simulink model "PeakDetect_500"  (R2018b)
settings: Solver=FixedStepAuto  StartTime=0  StopTime=500*(15e-9)  FixedStep=15e-9  RelTol=1e-3
libraries: simulink x35, hdlsllib x34
(part 3 of 3)

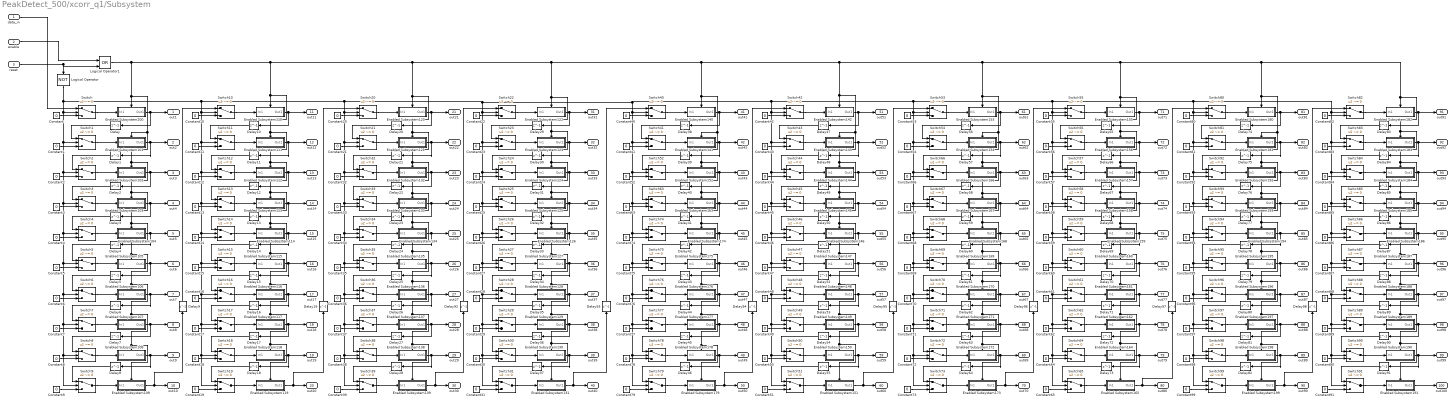
== system PeakDetect_500/xcorr_q1/Subsystem ==
  data_in : Inport  OutDataTypeStr=fixdt(1,16,15)
  enable : Inport  Port=2
  reset : Inport  Port=3
  Constant{,1..99} (100 alike) : Constant  Value=0  OutDataTypeStr=Inherit: Inherit via back propagation  SampleTime=-1
  Delay{,1..98} (99 alike) : Delay  DelayLength=1
  Enabled Subsystem101 : Subsystem  TreatAsAtomicUnit=on
  Enabled Subsystem102 : Subsystem  TreatAsAtomicUnit=on
  Enabled Subsystem103 : Subsystem  TreatAsAtomicUnit=on
  Enabled Subsystem104 : Subsystem  TreatAsAtomicUnit=on
  Enabled Subsystem105 : Subsystem  TreatAsAtomicUnit=on
  Enabled Subsystem106 : Subsystem  TreatAsAtomicUnit=on
  Enabled Subsystem107 : Subsystem  TreatAsAtomicUnit=on
  Enabled Subsystem108 : Subsystem  TreatAsAtomicUnit=on
  Enabled Subsystem109 : Subsystem  TreatAsAtomicUnit=on
  Enabled Subsystem110 : Subsystem  TreatAsAtomicUnit=on
  Enabled Subsystem111 : Subsystem  TreatAsAtomicUnit=on
  Enabled Subsystem112 : Subsystem  TreatAsAtomicUnit=on
  Enabled Subsystem113 : Subsystem  TreatAsAtomicUnit=on
  Enabled Subsystem114 : Subsystem  TreatAsAtomicUnit=on
  Enabled Subsystem115 : Subsystem  TreatAsAtomicUnit=on
  Enabled Subsystem116 : Subsystem  TreatAsAtomicUnit=on
  Enabled Subsystem117 : Subsystem  TreatAsAtomicUnit=on
  Enabled Subsystem118 : Subsystem  TreatAsAtomicUnit=on
  Enabled Subsystem119 : Subsystem  TreatAsAtomicUnit=on
  Enabled Subsystem120 : Subsystem  TreatAsAtomicUnit=on
  Enabled Subsystem121 : Subsystem  TreatAsAtomicUnit=on
  Enabled Subsystem122 : Subsystem  TreatAsAtomicUnit=on
  Enabled Subsystem123 : Subsystem  TreatAsAtomicUnit=on
  Enabled Subsystem124 : Subsystem  TreatAsAtomicUnit=on
  Enabled Subsystem125 : Subsystem  TreatAsAtomicUnit=on
  Enabled Subsystem126 : Subsystem  TreatAsAtomicUnit=on
  Enabled Subsystem127 : Subsystem  TreatAsAtomicUnit=on
  Enabled Subsystem128 : Subsystem  TreatAsAtomicUnit=on
  Enabled Subsystem129 : Subsystem  TreatAsAtomicUnit=on
  Enabled Subsystem130 : Subsystem  TreatAsAtomicUnit=on
  Enabled Subsystem131 : Subsystem  TreatAsAtomicUnit=on
  Enabled Subsystem132 : Subsystem  TreatAsAtomicUnit=on
  Enabled Subsystem133 : Subsystem  TreatAsAtomicUnit=on
  Enabled Subsystem134 : Subsystem  TreatAsAtomicUnit=on
  Enabled Subsystem135 : Subsystem  TreatAsAtomicUnit=on
  Enabled Subsystem136 : Subsystem  TreatAsAtomicUnit=on
  Enabled Subsystem137 : Subsystem  TreatAsAtomicUnit=on
  Enabled Subsystem138 : Subsystem  TreatAsAtomicUnit=on
  Enabled Subsystem139 : Subsystem  TreatAsAtomicUnit=on
  Enabled Subsystem140 : Subsystem  TreatAsAtomicUnit=on
  Enabled Subsystem141 : Subsystem  TreatAsAtomicUnit=on
  Enabled Subsystem142 : Subsystem  TreatAsAtomicUnit=on
  Enabled Subsystem143 : Subsystem  TreatAsAtomicUnit=on
  Enabled Subsystem144 : Subsystem  TreatAsAtomicUnit=on
  Enabled Subsystem145 : Subsystem  TreatAsAtomicUnit=on
  Enabled Subsystem146 : Subsystem  TreatAsAtomicUnit=on
  Enabled Subsystem147 : Subsystem  TreatAsAtomicUnit=on
  Enabled Subsystem148 : Subsystem  TreatAsAtomicUnit=on
  Enabled Subsystem149 : Subsystem  TreatAsAtomicUnit=on
  Enabled Subsystem150 : Subsystem  TreatAsAtomicUnit=on
  Enabled Subsystem151 : Subsystem  TreatAsAtomicUnit=on
  Enabled Subsystem152 : Subsystem  TreatAsAtomicUnit=on
  Enabled Subsystem153 : Subsystem  TreatAsAtomicUnit=on
  Enabled Subsystem154 : Subsystem  TreatAsAtomicUnit=on
  Enabled Subsystem155 : Subsystem  TreatAsAtomicUnit=on
  Enabled Subsystem156 : Subsystem  TreatAsAtomicUnit=on
  Enabled Subsystem157 : Subsystem  TreatAsAtomicUnit=on
  Enabled Subsystem158 : Subsystem  TreatAsAtomicUnit=on
  Enabled Subsystem159 : Subsystem  TreatAsAtomicUnit=on
  Enabled Subsystem160 : Subsystem  TreatAsAtomicUnit=on
  Enabled Subsystem161 : Subsystem  TreatAsAtomicUnit=on
  Enabled Subsystem162 : Subsystem  TreatAsAtomicUnit=on
  Enabled Subsystem163 : Subsystem  TreatAsAtomicUnit=on
  Enabled Subsystem164 : Subsystem  TreatAsAtomicUnit=on
  Enabled Subsystem165 : Subsystem  TreatAsAtomicUnit=on
  Enabled Subsystem166 : Subsystem  TreatAsAtomicUnit=on
  Enabled Subsystem167 : Subsystem  TreatAsAtomicUnit=on
  Enabled Subsystem168 : Subsystem  TreatAsAtomicUnit=on
  Enabled Subsystem169 : Subsystem  TreatAsAtomicUnit=on
  Enabled Subsystem170 : Subsystem  TreatAsAtomicUnit=on
  Enabled Subsystem171 : Subsystem  TreatAsAtomicUnit=on
  Enabled Subsystem172 : Subsystem  TreatAsAtomicUnit=on
  Enabled Subsystem173 : Subsystem  TreatAsAtomicUnit=on
  Enabled Subsystem174 : Subsystem  TreatAsAtomicUnit=on
  Enabled Subsystem175 : Subsystem  TreatAsAtomicUnit=on
  Enabled Subsystem176 : Subsystem  TreatAsAtomicUnit=on
  Enabled Subsystem177 : Subsystem  TreatAsAtomicUnit=on
  Enabled Subsystem178 : Subsystem  TreatAsAtomicUnit=on
  Enabled Subsystem179 : Subsystem  TreatAsAtomicUnit=on
  Enabled Subsystem180 : Subsystem  TreatAsAtomicUnit=on
  Enabled Subsystem181 : Subsystem  TreatAsAtomicUnit=on
  Enabled Subsystem182 : Subsystem  TreatAsAtomicUnit=on
  Enabled Subsystem183 : Subsystem  TreatAsAtomicUnit=on
  Enabled Subsystem184 : Subsystem  TreatAsAtomicUnit=on
  Enabled Subsystem185 : Subsystem  TreatAsAtomicUnit=on
  Enabled Subsystem186 : Subsystem  TreatAsAtomicUnit=on
  Enabled Subsystem187 : Subsystem  TreatAsAtomicUnit=on
  Enabled Subsystem188 : Subsystem  TreatAsAtomicUnit=on
  Enabled Subsystem189 : Subsystem  TreatAsAtomicUnit=on
  Enabled Subsystem190 : Subsystem  TreatAsAtomicUnit=on
  Enabled Subsystem191 : Subsystem  TreatAsAtomicUnit=on
  Enabled Subsystem192 : Subsystem  TreatAsAtomicUnit=on
  Enabled Subsystem193 : Subsystem  TreatAsAtomicUnit=on
  Enabled Subsystem194 : Subsystem  TreatAsAtomicUnit=on
  Enabled Subsystem195 : Subsystem  TreatAsAtomicUnit=on
  Enabled Subsystem196 : Subsystem  TreatAsAtomicUnit=on
  Enabled Subsystem197 : Subsystem  TreatAsAtomicUnit=on
  Enabled Subsystem198 : Subsystem  TreatAsAtomicUnit=on
  Enabled Subsystem199 : Subsystem  TreatAsAtomicUnit=on
  Enabled Subsystem200 : Subsystem  TreatAsAtomicUnit=on
  Logical Operator : Logic  Operator=NOT  IconShape=distinctive  AllPortsSameDT=off  OutDataTypeStr=boolean
  Logical Operator1 : Logic  Operator=OR  IconShape=distinctive  AllPortsSameDT=off  OutDataTypeStr=boolean
  Switch{,1..99} (100 alike) : Switch  Criteria=u2 ~= 0  OutDataTypeStr=Inherit: Inherit via back propagation
  out1 : Outport
  out2 : Outport  Port=2
  out3 : Outport  Port=3
  out4 : Outport  Port=4
  out5 : Outport  Port=5
  out6 : Outport  Port=6
  out7 : Outport  Port=7
  out8 : Outport  Port=8
  out9 : Outport  Port=9
  out10 : Outport  Port=10
  out11 : Outport  Port=11
  out12 : Outport  Port=12
  out13 : Outport  Port=13
  out14 : Outport  Port=14
  out15 : Outport  Port=15
  out16 : Outport  Port=16
  out17 : Outport  Port=17
  out18 : Outport  Port=18
  out19 : Outport  Port=19
  out20 : Outport  Port=20
  out21 : Outport  Port=21
  out22 : Outport  Port=22
  out23 : Outport  Port=23
  out24 : Outport  Port=24
  out25 : Outport  Port=25
  out26 : Outport  Port=26
  out27 : Outport  Port=27
  out28 : Outport  Port=28
  out29 : Outport  Port=29
  out30 : Outport  Port=30
  out31 : Outport  Port=31
  out32 : Outport  Port=32
  out33 : Outport  Port=33
  out34 : Outport  Port=34
  out35 : Outport  Port=35
  out36 : Outport  Port=36
  out37 : Outport  Port=37
  out38 : Outport  Port=38
  out39 : Outport  Port=39
  out40 : Outport  Port=40
  out41 : Outport  Port=41
  out42 : Outport  Port=42
  out43 : Outport  Port=43
  out44 : Outport  Port=44
  out45 : Outport  Port=45
  out46 : Outport  Port=46
  out47 : Outport  Port=47
  out48 : Outport  Port=48
  out49 : Outport  Port=49
  out50 : Outport  Port=50
  out51 : Outport  Port=51
  out52 : Outport  Port=52
  out53 : Outport  Port=53
  out54 : Outport  Port=54
  out55 : Outport  Port=55
  out56 : Outport  Port=56
  out57 : Outport  Port=57
  out58 : Outport  Port=58
  out59 : Outport  Port=59
  out60 : Outport  Port=60
  out61 : Outport  Port=61
  out62 : Outport  Port=62
  out63 : Outport  Port=63
  out64 : Outport  Port=64
  out65 : Outport  Port=65
  out66 : Outport  Port=66
  out67 : Outport  Port=67
  out68 : Outport  Port=68
  out69 : Outport  Port=69
  out70 : Outport  Port=70
  out71 : Outport  Port=71
  out72 : Outport  Port=72
  out73 : Outport  Port=73
  out74 : Outport  Port=74
  out75 : Outport  Port=75
  out76 : Outport  Port=76
  out77 : Outport  Port=77
  out78 : Outport  Port=78
  out79 : Outport  Port=79
  out80 : Outport  Port=80
  out81 : Outport  Port=81
  out82 : Outport  Port=82
  out83 : Outport  Port=83
  out84 : Outport  Port=84
  out85 : Outport  Port=85
  out86 : Outport  Port=86
  out87 : Outport  Port=87
  out88 : Outport  Port=88
  out89 : Outport  Port=89
  out90 : Outport  Port=90
  out91 : Outport  Port=91
  out92 : Outport  Port=92
  out93 : Outport  Port=93
  out94 : Outport  Port=94
  out95 : Outport  Port=95
  out96 : Outport  Port=96
  out97 : Outport  Port=97
  out98 : Outport  Port=98
  out99 : Outport  Port=99
  out100 : Outport  Port=100
  wires:
  Delay81/1 -> Switch98/1
  Delay36/1 -> Switch30/1
  Constant37/1 -> Switch37/3
  Switch72/1 -> Enabled Subsystem172/1(In1)
  Switch33/1 -> Enabled Subsystem133/1(In1)
  Delay65/1 -> Switch56/1
  Constant39/1 -> Switch39/3
  Switch76/1 -> Enabled Subsystem176/1(In1)
  Constant59/1 -> Switch59/3
  Constant70/1 -> Switch70/3
  Constant12/1 -> Switch12/3
  Constant58/1 -> Switch58/3
  Delay52/1 -> Switch48/1
  Switch58/1 -> Enabled Subsystem158/1(In1)
  Constant55/1 -> Switch55/3
  Switch29/1 -> Enabled Subsystem129/1(In1)
  Switch37/1 -> Enabled Subsystem137/1(In1)
  Constant99/1 -> Switch99/3
  Constant22/1 -> Switch22/3
  Constant34/1 -> Switch34/3
  Switch38/1 -> Enabled Subsystem138/1(In1)
  Delay/1 -> Switch1/1
  Switch23/1 -> Enabled Subsystem123/1(In1)
  Delay25/1 -> Switch36/1
  Delay22/1 -> Switch33/1
  Delay50/1 -> Switch46/1
  Constant53/1 -> Switch53/3
  Enabled Subsystem197/1(Out1) -> out88/1, Delay81/1
  Switch45/1 -> Enabled Subsystem145/1(In1)
  Switch6/1 -> Enabled Subsystem106/1(In1)
  Delay92/1 -> Switch22/1
  Switch55/1 -> Enabled Subsystem155/1(In1)
  Constant38/1 -> Switch38/3
  Delay58/1 -> Switch67/1
  Enabled Subsystem176/1(Out1) -> out47/1, Delay44/1
  Constant54/1 -> Switch54/3
  Constant31/1 -> Switch31/3
  Enabled Subsystem139/1(Out1) -> out30/1, Delay92/1
  Delay94/1 -> Switch42/1
  Switch90/1 -> Enabled Subsystem190/1(In1)
  Delay8/1 -> Switch9/1
  Constant50/1 -> Switch50/3
  Enabled Subsystem155/1(Out1) -> out71/1, Delay65/1
  Delay72/1 -> Switch64/1
  Constant76/1 -> Switch76/3
  Switch73/1 -> Enabled Subsystem173/1(In1)
  Constant41/1 -> Switch41/3
  Constant97/1 -> Switch97/3
  Switch44/1 -> Enabled Subsystem144/1(In1)
  Switch77/1 -> Enabled Subsystem177/1(In1)
  Constant47/1 -> Switch47/3
  Constant62/1 -> Switch62/3
  Switch3/1 -> Enabled Subsystem103/1(In1)
  Constant71/1 -> Switch71/3
  Delay37/1 -> Switch31/1
  Constant75/1 -> Switch75/3
  Constant93/1 -> Switch93/3
  Switch2/1 -> Enabled Subsystem102/1(In1)
  Constant29/1 -> Switch29/3
  Enabled Subsystem172/1(Out1) -> out69/1, Delay64/1
  Delay24/1 -> Switch35/1
  Constant56/1 -> Switch56/3
  Switch8/1 -> Enabled Subsystem108/1(In1)
  Switch31/1 -> Enabled Subsystem131/1(In1)
  Delay89/1 -> Switch89/1
  Delay27/1 -> Switch38/1
  Constant2/1 -> Switch2/3
  Switch13/1 -> Enabled Subsystem113/1(In1)
  Constant/1 -> Switch/3
  Delay64/1 -> Switch73/1
  Constant81/1 -> Switch81/3
  Constant40/1 -> Switch40/3
  Switch52/1 -> Enabled Subsystem152/1(In1)
  Switch14/1 -> Enabled Subsystem114/1(In1)
  Enabled Subsystem117/1(Out1) -> out18/1, Delay17/1
  Constant49/1 -> Switch49/3
  Switch70/1 -> Enabled Subsystem170/1(In1)
  Constant64/1 -> Switch64/3
  Switch82/1 -> Enabled Subsystem182/1(In1)
  Delay98/1 -> Switch82/1
  Enabled Subsystem177/1(Out1) -> out48/1, Delay45/1
  Enabled Subsystem159/1(Out1) -> out75/1, Delay69/1
  Constant68/1 -> Switch68/3
  Enabled Subsystem101/1(Out1) -> out2/1, Delay1/1
  Constant92/1 -> Switch92/3
  Enabled Subsystem152/1(Out1) -> out43/1, Delay40/1
  Enabled Subsystem136/1(Out1) -> out27/1, Delay26/1
  Delay86/1 -> Switch86/1
  Constant83/1 -> Switch83/3
  Switch83/1 -> Enabled Subsystem183/1(In1)
  Enabled Subsystem163/1(Out1) -> out44/1, Delay41/1
  Switch15/1 -> Enabled Subsystem115/1(In1)
  Constant46/1 -> Switch46/3
  Delay39/1 -> Switch52/1
  Delay31/1 -> Switch25/1
  Constant6/1 -> Switch6/3
  Switch26/1 -> Enabled Subsystem126/1(In1)
  Delay29/1 -> Switch23/1
  Constant28/1 -> Switch28/3
  Constant11/1 -> Switch11/3
  Constant9/1 -> Switch9/3
  Enabled Subsystem105/1(Out1) -> out6/1, Delay5/1
  Delay48/1 -> Switch44/1
  Switch4/1 -> Enabled Subsystem104/1(In1)
  Delay77/1 -> Switch94/1
  Constant24/1 -> Switch24/3
  Switch17/1 -> Enabled Subsystem117/1(In1)
  Switch32/1 -> Enabled Subsystem132/1(In1)
  Enabled Subsystem149/1(Out1) -> out58/1, Delay54/1
  Constant73/1 -> Switch73/3
  Switch34/1 -> Enabled Subsystem134/1(In1)
  Delay76/1 -> Switch93/1
  Enabled Subsystem148/1(Out1) -> out57/1, Delay53/1
  Switch74/1 -> Enabled Subsystem174/1(In1)
  Enabled Subsystem153/1(Out1) -> out61/1, Delay56/1
  Enabled Subsystem144/1(Out1) -> out53/1, Delay49/1
  Delay90/1 -> Switch90/1
  Constant61/1 -> Switch61/3
  Switch63/1 -> Enabled Subsystem163/1(In1)
  Switch89/1 -> Enabled Subsystem189/1(In1)
  Switch94/1 -> Enabled Subsystem194/1(In1)
  Delay67/1 -> Switch58/1
  Constant19/1 -> Switch19/3
  Switch65/1 -> Enabled Subsystem165/1(In1)
  Constant4/1 -> Switch4/3
  Constant96/1 -> Switch96/3
  Enabled Subsystem167/1(Out1) -> out64/1, Delay59/1
  Delay75/1 -> Switch92/1
  Delay11/1 -> Switch12/1
  Constant51/1 -> Switch51/3
  Enabled Subsystem111/1(Out1) -> out12/1, Delay11/1
  Switch11/1 -> Enabled Subsystem111/1(In1)
  Constant94/1 -> Switch94/3
  Switch28/1 -> Enabled Subsystem128/1(In1)
  Constant80/1 -> Switch80/3
  Constant74/1 -> Switch74/3
  Switch27/1 -> Enabled Subsystem127/1(In1)
  Enabled Subsystem110/1(Out1) -> out11/1, Delay10/1
  Delay97/1 -> Switch80/1
  Enabled Subsystem200/1(Out1) -> out1/1, Delay/1
  Switch95/1 -> Enabled Subsystem195/1(In1)
  Switch99/1 -> Enabled Subsystem199/1(In1)
  Switch12/1 -> Enabled Subsystem112/1(In1)
  Switch19/1 -> Enabled Subsystem119/1(In1)
  Switch36/1 -> Enabled Subsystem136/1(In1)
  Constant87/1 -> Switch87/3
  Delay7/1 -> Switch8/1
  Constant30/1 -> Switch30/3
  Enabled Subsystem150/1(Out1) -> out59/1, Delay55/1
  Switch51/1 -> Enabled Subsystem151/1(In1)
  Constant33/1 -> Switch33/3
  Enabled Subsystem160/1(Out1) -> out76/1, Delay70/1
  Delay28/1 -> Switch39/1
  Enabled Subsystem154/1(Out1) -> out62/1, Delay57/1
  Delay41/1 -> Switch74/1
  Delay3/1 -> Switch4/1
  Constant8/1 -> Switch8/3
  Constant72/1 -> Switch72/3
  Switch61/1 -> Enabled Subsystem161/1(In1)
  Constant18/1 -> Switch18/3
  Delay79/1 -> Switch96/1
  Enabled Subsystem193/1(Out1) -> out84/1, Delay77/1
  Delay88/1 -> Switch88/1
  Constant67/1 -> Switch67/3
  Switch97/1 -> Enabled Subsystem197/1(In1)
  data_in/1 -> Switch/1
  Enabled Subsystem113/1(Out1) -> out14/1, Delay13/1
  Constant82/1 -> Switch82/3
  Constant15/1 -> Switch15/3
  Switch93/1 -> Enabled Subsystem193/1(In1)
  Delay61/1 -> Switch70/1
  Logical Operator/1 -> Switch91/2, Switch90/2, Switch89/2, Switch88/2, Switch87/2, Switch86/2, Switch85/2, Switch84/2, Switch83/2, Switch82/2, Switch99/2, Switch98/2, Switch97/2, Switch96/2, Switch95/2, Switch94/2, Switch93/2, Switch92/2, Switch81/2, Switch80/2, Switch65/2, Switch64/2, Switch62/2, Switch61/2, Switch60/2, Switch59/2, Switch58/2, Switch57/2, Switch56/2, Switch55/2, Switch73/2, Switch72/2, Switch71/2, Switch70/2, Switch69/2, Switch68/2, Switch67/2, Switch66/2, Switch54/2, Switch53/2, Switch51/2, Switch50/2, Switch49/2, Switch48/2, Switch47/2, Switch46/2, Switch45/2, Switch44/2, Switch43/2, Switch42/2, Switch79/2, Switch78/2, Switch77/2, Switch76/2, Switch75/2, Switch74/2, Switch63/2, Switch52/2, Switch41/2, Switch40/2, Switch31/2, Switch30/2, Switch29/2, Switch28/2, Switch27/2, Switch26/2, Switch25/2, Switch24/2, Switch23/2, Switch22/2, Switch39/2, Switch38/2, Switch37/2, Switch36/2, Switch35/2, Switch34/2, Switch33/2, Switch32/2, Switch21/2, Switch20/2, Switch19/2, Switch18/2, Switch17/2, Switch16/2, Switch15/2, Switch14/2, Switch13/2, Switch12/2, Switch11/2, Switch10/2, Switch9/2, Switch8/2, Switch7/2, Switch6/2, Switch5/2, Switch4/2, Switch3/2, Switch2/2, Switch1/2, Switch/2
  Delay85/1 -> Switch85/1
  Switch25/1 -> Enabled Subsystem125/1(In1)
  Enabled Subsystem118/1(Out1) -> out19/1, Delay18/1
  Enabled Subsystem129/1(Out1) -> out38/1, Delay36/1
  Switch80/1 -> Enabled Subsystem180/1(In1)
  Enabled Subsystem112/1(Out1) -> out13/1, Delay12/1
  Enabled Subsystem120/1(Out1) -> out21/1, Delay20/1
  Switch21/1 -> Enabled Subsystem121/1(In1)
  Delay18/1 -> Switch19/1
  Enabled Subsystem134/1(Out1) -> out25/1, Delay24/1
  Enabled Subsystem147/1(Out1) -> out56/1, Delay52/1
  Constant86/1 -> Switch86/3
  Constant35/1 -> Switch35/3
  Delay9/1 -> Switch10/1
  Constant13/1 -> Switch13/3
  Delay93/1 -> Switch40/1
  Enabled Subsystem166/1(Out1) -> out63/1, Delay58/1
  Delay59/1 -> Switch68/1
  Enabled Subsystem157/1(Out1) -> out73/1, Delay67/1
  Switch88/1 -> Enabled Subsystem188/1(In1)
  Constant66/1 -> Switch66/3
  Delay32/1 -> Switch26/1
  Constant88/1 -> Switch88/3
  Enabled Subsystem130/1(Out1) -> out39/1, Delay37/1
  Switch79/1 -> Enabled Subsystem179/1(In1)
  Constant89/1 -> Switch89/3
  Enabled Subsystem161/1(Out1) -> out77/1, Delay71/1
  Delay16/1 -> Switch17/1
  Switch56/1 -> Enabled Subsystem156/1(In1)
  Enabled Subsystem185/1(Out1) -> out94/1, Delay86/1
  Enabled Subsystem164/1(Out1) -> out79/1, Delay73/1
  Delay71/1 -> Switch62/1
  Enabled Subsystem180/1(Out1) -> out81/1, Delay74/1
  Enabled Subsystem171/1(Out1) -> out68/1, Delay63/1
  Enabled Subsystem184/1(Out1) -> out93/1, Delay85/1
  Enabled Subsystem107/1(Out1) -> out8/1, Delay7/1
  Switch75/1 -> Enabled Subsystem175/1(In1)
  Switch18/1 -> Enabled Subsystem118/1(In1)
  Delay38/1 -> Switch41/1
  Constant85/1 -> Switch85/3
  Switch47/1 -> Enabled Subsystem147/1(In1)
  Constant91/1 -> Switch91/3
  Constant26/1 -> Switch26/3
  Delay2/1 -> Switch3/1
  Delay57/1 -> Switch66/1
  Constant20/1 -> Switch20/3
  Delay82/1 -> Switch99/1
  Enabled Subsystem122/1(Out1) -> out31/1, Delay29/1
  Delay70/1 -> Switch61/1
  Delay33/1 -> Switch27/1
  Constant60/1 -> Switch60/3
  Delay95/1 -> Switch53/1
  Constant32/1 -> Switch32/3
  Switch87/1 -> Enabled Subsystem187/1(In1)
  Enabled Subsystem182/1(Out1) -> out91/1, Delay83/1
  Switch92/1 -> Enabled Subsystem192/1(In1)
  Delay13/1 -> Switch14/1
  Delay47/1 -> Switch43/1
  Constant98/1 -> Switch98/3
  Switch81/1 -> Enabled Subsystem181/1(In1)
  Delay96/1 -> Switch55/1
  Delay35/1 -> Switch29/1
  Delay73/1 -> Switch65/1
  Enabled Subsystem196/1(Out1) -> out87/1, Delay80/1
  Enabled Subsystem103/1(Out1) -> out4/1, Delay3/1
  Constant23/1 -> Switch23/3
  Constant90/1 -> Switch90/3
  Enabled Subsystem125/1(Out1) -> out34/1, Delay32/1
  Enabled Subsystem169/1(Out1) -> out66/1, Delay61/1
  Constant78/1 -> Switch78/3
  Constant27/1 -> Switch27/3
  Delay14/1 -> Switch15/1
  Enabled Subsystem104/1(Out1) -> out5/1, Delay4/1
  Constant36/1 -> Switch36/3
  Switch39/1 -> Enabled Subsystem139/1(In1)
  Delay42/1 -> Switch75/1
  Enabled Subsystem114/1(Out1) -> out15/1, Delay14/1
  Enabled Subsystem146/1(Out1) -> out55/1, Delay51/1
  Switch57/1 -> Enabled Subsystem157/1(In1)
  Delay87/1 -> Switch87/1
  Enabled Subsystem137/1(Out1) -> out28/1, Delay27/1
  Constant84/1 -> Switch84/3
  Constant1/1 -> Switch1/3
  Enabled Subsystem173/1(Out1) -> out70/1, Delay96/1
  Switch41/1 -> Enabled Subsystem141/1(In1)
  Delay20/1 -> Switch21/1
  Delay68/1 -> Switch59/1
  Switch98/1 -> Enabled Subsystem198/1(In1)
  Delay43/1 -> Switch76/1
  Constant65/1 -> Switch65/3
  Constant17/1 -> Switch17/3
  Switch60/1 -> Enabled Subsystem160/1(In1)
  Enabled Subsystem162/1(Out1) -> out78/1, Delay72/1
  Constant7/1 -> Switch7/3
  Delay78/1 -> Switch95/1
  Enabled Subsystem191/1(Out1) -> out100/1
  Switch40/1 -> Enabled Subsystem140/1(In1)
  Switch78/1 -> Enabled Subsystem178/1(In1)
  Switch85/1 -> Enabled Subsystem185/1(In1)
  Delay12/1 -> Switch13/1
  Switch86/1 -> Enabled Subsystem186/1(In1)
  Delay84/1 -> Switch84/1
  Constant77/1 -> Switch77/3
  Delay6/1 -> Switch7/1
  Constant42/1 -> Switch42/3
  Delay80/1 -> Switch97/1
  Delay53/1 -> Switch49/1
  Enabled Subsystem128/1(Out1) -> out37/1, Delay35/1
  Enabled Subsystem170/1(Out1) -> out67/1, Delay62/1
  Enabled Subsystem102/1(Out1) -> out3/1, Delay2/1
  Enabled Subsystem194/1(Out1) -> out85/1, Delay78/1
  Constant10/1 -> Switch10/3
  Enabled Subsystem187/1(Out1) -> out96/1, Delay88/1
  enable/1 -> Logical Operator1/1
  Enabled Subsystem123/1(Out1) -> out32/1, Delay30/1
  Delay26/1 -> Switch37/1
  Switch62/1 -> Enabled Subsystem162/1(In1)
  Enabled Subsystem141/1(Out1) -> out42/1, Delay39/1
  Delay83/1 -> Switch83/1
  Delay45/1 -> Switch78/1
  Switch10/1 -> Enabled Subsystem110/1(In1)
  Enabled Subsystem138/1(Out1) -> out29/1, Delay28/1
  Enabled Subsystem192/1(Out1) -> out83/1, Delay76/1
  Delay5/1 -> Switch6/1
  Switch53/1 -> Enabled Subsystem153/1(In1)
  Enabled Subsystem126/1(Out1) -> out35/1, Delay33/1
  Switch48/1 -> Enabled Subsystem148/1(In1)
  Delay55/1 -> Switch51/1
  Delay34/1 -> Switch28/1
  Switch7/1 -> Enabled Subsystem107/1(In1)
  Enabled Subsystem186/1(Out1) -> out95/1, Delay87/1
  Delay10/1 -> Switch11/1
  Enabled Subsystem199/1(Out1) -> out90/1, Delay98/1
  Constant52/1 -> Switch52/3
  Switch96/1 -> Enabled Subsystem196/1(In1)
  Constant44/1 -> Switch44/3
  Delay69/1 -> Switch60/1
  Enabled Subsystem131/1(Out1) -> out40/1, Delay93/1
  Enabled Subsystem179/1(Out1) -> out50/1, Delay94/1
  Switch46/1 -> Enabled Subsystem146/1(In1)
  Delay30/1 -> Switch24/1
  Enabled Subsystem133/1(Out1) -> out24/1, Delay23/1
  Enabled Subsystem109/1(Out1) -> out10/1, Delay9/1
  Enabled Subsystem119/1(Out1) -> out20/1, Delay19/1
  Switch5/1 -> Enabled Subsystem105/1(In1)
  Constant69/1 -> Switch69/3
  Enabled Subsystem142/1(Out1) -> out51/1, Delay47/1
  Delay17/1 -> Switch18/1
  Constant45/1 -> Switch45/3
  Delay46/1 -> Switch79/1
  Enabled Subsystem181/1(Out1) -> out82/1, Delay75/1
  Enabled Subsystem135/1(Out1) -> out26/1, Delay25/1
  Enabled Subsystem124/1(Out1) -> out33/1, Delay31/1
  Delay15/1 -> Switch16/1
  Delay54/1 -> Switch50/1
  Enabled Subsystem183/1(Out1) -> out92/1, Delay84/1
  Constant57/1 -> Switch57/3
  Delay49/1 -> Switch45/1
  Delay74/1 -> Switch81/1
  Delay4/1 -> Switch5/1
  Enabled Subsystem143/1(Out1) -> out52/1, Delay48/1
  Switch67/1 -> Enabled Subsystem167/1(In1)
  Constant5/1 -> Switch5/3
  Switch42/1 -> Enabled Subsystem142/1(In1)
  Constant14/1 -> Switch14/3
  Switch91/1 -> Enabled Subsystem191/1(In1)
  Enabled Subsystem145/1(Out1) -> out54/1, Delay50/1
  Delay63/1 -> Switch72/1
  Delay44/1 -> Switch77/1
  Delay60/1 -> Switch69/1
  Switch50/1 -> Enabled Subsystem150/1(In1)
  Enabled Subsystem121/1(Out1) -> out22/1, Delay21/1
  Delay19/1 -> Switch20/1
  reset/1 -> Logical Operator1/2, Logical Operator/1
  Constant43/1 -> Switch43/3
  Delay40/1 -> Switch63/1
  Enabled Subsystem140/1(Out1) -> out41/1, Delay38/1
  Switch69/1 -> Enabled Subsystem169/1(In1)
  Enabled Subsystem151/1(Out1) -> out60/1, Delay95/1
  Delay91/1 -> Switch91/1
  Constant25/1 -> Switch25/3
  Delay21/1 -> Switch32/1
  Enabled Subsystem195/1(Out1) -> out86/1, Delay79/1
  Enabled Subsystem132/1(Out1) -> out23/1, Delay22/1
  Delay51/1 -> Switch47/1
  Switch20/1 -> Enabled Subsystem120/1(In1)
  Switch84/1 -> Enabled Subsystem184/1(In1)
  Switch9/1 -> Enabled Subsystem109/1(In1)
  Delay62/1 -> Switch71/1
  Enabled Subsystem127/1(Out1) -> out36/1, Delay34/1
  Enabled Subsystem190/1(Out1) -> out99/1, Delay91/1
  Switch54/1 -> Enabled Subsystem154/1(In1)
  Enabled Subsystem198/1(Out1) -> out89/1, Delay82/1
  Delay66/1 -> Switch57/1
  Switch22/1 -> Enabled Subsystem122/1(In1)
  Switch68/1 -> Enabled Subsystem168/1(In1)
  Delay56/1 -> Switch54/1
  Constant95/1 -> Switch95/3
  Switch24/1 -> Enabled Subsystem124/1(In1)
  Enabled Subsystem106/1(Out1) -> out7/1, Delay6/1
  Constant3/1 -> Switch3/3
  Enabled Subsystem189/1(Out1) -> out98/1, Delay90/1
  Switch16/1 -> Enabled Subsystem116/1(In1)
  Switch49/1 -> Enabled Subsystem149/1(In1)
  Enabled Subsystem158/1(Out1) -> out74/1, Delay68/1
  Switch71/1 -> Enabled Subsystem171/1(In1)
  Switch64/1 -> Enabled Subsystem164/1(In1)
  Enabled Subsystem175/1(Out1) -> out46/1, Delay43/1
  Logical Operator1/1 -> Enabled Subsystem200/Enable, Enabled Subsystem101/Enable, Enabled Subsystem109/Enable, Enabled Subsystem108/Enable, Enabled Subsystem107/Enable, Enabled Subsystem106/Enable, Enabled Subsystem105/Enable, Enabled Subsystem104/Enable, Enabled Subsystem103/Enable, Enabled Subsystem102/Enable, Enabled Subsystem181/Enable, Enabled Subsystem199/Enable, Enabled Subsystem198/Enable, Enabled Subsystem197/Enable, Enabled Subsystem196/Enable, Enabled Subsystem195/Enable, Enabled Subsystem194/Enable, Enabled Subsystem193/Enable, Enabled Subsystem192/Enable, Enabled Subsystem180/Enable, Enabled Subsystem191/Enable, Enabled Subsystem190/Enable, Enabled Subsystem189/Enable, Enabled Subsystem188/Enable, Enabled Subsystem187/Enable, Enabled Subsystem186/Enable, Enabled Subsystem185/Enable, Enabled Subsystem184/Enable, Enabled Subsystem183/Enable, Enabled Subsystem182/Enable, Enabled Subsystem165/Enable, Enabled Subsystem164/Enable, Enabled Subsystem162/Enable, Enabled Subsystem161/Enable, Enabled Subsystem160/Enable, Enabled Subsystem159/Enable, Enabled Subsystem158/Enable, Enabled Subsystem157/Enable, Enabled Subsystem156/Enable, Enabled Subsystem155/Enable, Enabled Subsystem154/Enable, Enabled Subsystem173/Enable, Enabled Subsystem172/Enable, Enabled Subsystem171/Enable, Enabled Subsystem170/Enable, Enabled Subsystem169/Enable, Enabled Subsystem168/Enable, Enabled Subsystem167/Enable, Enabled Subsystem166/Enable, Enabled Subsystem153/Enable, Enabled Subsystem143/Enable, Enabled Subsystem151/Enable, Enabled Subsystem150/Enable, Enabled Subsystem149/Enable, Enabled Subsystem148/Enable, Enabled Subsystem147/Enable, Enabled Subsystem146/Enable, Enabled Subsystem145/Enable, Enabled Subsystem144/Enable, Enabled Subsystem142/Enable, Enabled Subsystem141/Enable, Enabled Subsystem179/Enable, Enabled Subsystem178/Enable, Enabled Subsystem177/Enable, Enabled Subsystem176/Enable, Enabled Subsystem175/Enable, Enabled Subsystem174/Enable, Enabled Subsystem163/Enable, Enabled Subsystem152/Enable, Enabled Subsystem140/Enable, Enabled Subsystem131/Enable, Enabled Subsystem130/Enable, Enabled Subsystem129/Enable, Enabled Subsystem128/Enable, Enabled Subsystem127/Enable, Enabled Subsystem126/Enable, Enabled Subsystem125/Enable, Enabled Subsystem124/Enable, Enabled Subsystem123/Enable, Enabled Subsystem122/Enable, Enabled Subsystem139/Enable, Enabled Subsystem138/Enable, Enabled Subsystem137/Enable, Enabled Subsystem136/Enable, Enabled Subsystem135/Enable, Enabled Subsystem134/Enable, Enabled Subsystem133/Enable, Enabled Subsystem132/Enable, Enabled Subsystem121/Enable, Enabled Subsystem120/Enable, Enabled Subsystem110/Enable, Enabled Subsystem119/Enable, Enabled Subsystem118/Enable, Enabled Subsystem117/Enable, Enabled Subsystem116/Enable, Enabled Subsystem115/Enable, Enabled Subsystem114/Enable, Enabled Subsystem113/Enable, Enabled Subsystem112/Enable, Enabled Subsystem111/Enable
  Constant16/1 -> Switch16/3
  Delay23/1 -> Switch34/1
  Switch1/1 -> Enabled Subsystem101/1(In1)
  Constant79/1 -> Switch79/3
  Switch/1 -> Enabled Subsystem200/1(In1)
  Switch30/1 -> Enabled Subsystem130/1(In1)
  Delay1/1 -> Switch2/1
  Enabled Subsystem115/1(Out1) -> out16/1, Delay15/1
  Enabled Subsystem156/1(Out1) -> out72/1, Delay66/1
  Enabled Subsystem178/1(Out1) -> out49/1, Delay46/1
  Enabled Subsystem168/1(Out1) -> out65/1, Delay60/1
  Constant48/1 -> Switch48/3
  Enabled Subsystem165/1(Out1) -> out80/1, Delay97/1
  Enabled Subsystem188/1(Out1) -> out97/1, Delay89/1
  Switch66/1 -> Enabled Subsystem166/1(In1)
  Enabled Subsystem108/1(Out1) -> out9/1, Delay8/1
  Switch59/1 -> Enabled Subsystem159/1(In1)
  Switch35/1 -> Enabled Subsystem135/1(In1)
  Constant21/1 -> Switch21/3
  Enabled Subsystem174/1(Out1) -> out45/1, Delay42/1
  Enabled Subsystem116/1(Out1) -> out17/1, Delay16/1
  Switch43/1 -> Enabled Subsystem143/1(In1)
  Constant63/1 -> Switch63/3

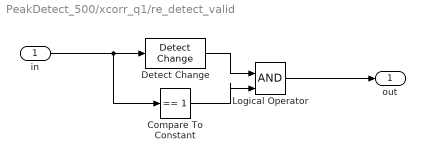
== system PeakDetect_500/xcorr_q1/re_detect_valid ==
  in : Inport  OutDataTypeStr=boolean
  Compare To Constant : simulink/Logic and Bit Operations/Compare To Constant  relop===  const=1  OutDataTypeStr=boolean
  Detect Change : simulink/Logic and Bit Operations/Detect Change  vinit=0  OutDataTypeStr=boolean
  Logical Operator : Logic  IconShape=distinctive  AllPortsSameDT=off  OutDataTypeStr=boolean
  out : Outport  OutDataTypeStr=boolean
  wires:
  Logical Operator/1 -> out/1
  Compare To Constant/1 -> Logical Operator/2
  Detect Change/1 -> Logical Operator/1
  in/1 -> Compare To Constant/1, Detect Change/1

== system PeakDetect_500/xcorr_q1/Subsystem/Enabled Subsystem101 ==
  In1 : Inport
  Enable : EnablePort
  Out1 : Outport  InitialOutput=0
  wires:
  In1/1 -> Out1/1

== system PeakDetect_500/xcorr_q1/Subsystem/Enabled Subsystem102 ==
  In1 : Inport
  Enable : EnablePort
  Out1 : Outport  InitialOutput=0
  wires:
  In1/1 -> Out1/1

== system PeakDetect_500/xcorr_q1/Subsystem/Enabled Subsystem103 ==
  In1 : Inport
  Enable : EnablePort
  Out1 : Outport  InitialOutput=0
  wires:
  In1/1 -> Out1/1

== system PeakDetect_500/xcorr_q1/Subsystem/Enabled Subsystem104 ==
  In1 : Inport
  Enable : EnablePort
  Out1 : Outport  InitialOutput=0
  wires:
  In1/1 -> Out1/1

== system PeakDetect_500/xcorr_q1/Subsystem/Enabled Subsystem105 ==
  In1 : Inport
  Enable : EnablePort
  Out1 : Outport  InitialOutput=0
  wires:
  In1/1 -> Out1/1

== system PeakDetect_500/xcorr_q1/Subsystem/Enabled Subsystem106 ==
  In1 : Inport
  Enable : EnablePort
  Out1 : Outport  InitialOutput=0
  wires:
  In1/1 -> Out1/1

== system PeakDetect_500/xcorr_q1/Subsystem/Enabled Subsystem107 ==
  In1 : Inport
  Enable : EnablePort
  Out1 : Outport  InitialOutput=0
  wires:
  In1/1 -> Out1/1

== system PeakDetect_500/xcorr_q1/Subsystem/Enabled Subsystem108 ==
  In1 : Inport
  Enable : EnablePort
  Out1 : Outport  InitialOutput=0
  wires:
  In1/1 -> Out1/1

== system PeakDetect_500/xcorr_q1/Subsystem/Enabled Subsystem109 ==
  In1 : Inport
  Enable : EnablePort
  Out1 : Outport  InitialOutput=0
  wires:
  In1/1 -> Out1/1

== system PeakDetect_500/xcorr_q1/Subsystem/Enabled Subsystem110 ==
  In1 : Inport
  Enable : EnablePort
  Out1 : Outport  InitialOutput=0
  wires:
  In1/1 -> Out1/1

== system PeakDetect_500/xcorr_q1/Subsystem/Enabled Subsystem111 ==
  In1 : Inport
  Enable : EnablePort
  Out1 : Outport  InitialOutput=0
  wires:
  In1/1 -> Out1/1

== system PeakDetect_500/xcorr_q1/Subsystem/Enabled Subsystem112 ==
  In1 : Inport
  Enable : EnablePort
  Out1 : Outport  InitialOutput=0
  wires:
  In1/1 -> Out1/1

== system PeakDetect_500/xcorr_q1/Subsystem/Enabled Subsystem113 ==
  In1 : Inport
  Enable : EnablePort
  Out1 : Outport  InitialOutput=0
  wires:
  In1/1 -> Out1/1

== system PeakDetect_500/xcorr_q1/Subsystem/Enabled Subsystem114 ==
  In1 : Inport
  Enable : EnablePort
  Out1 : Outport  InitialOutput=0
  wires:
  In1/1 -> Out1/1

== system PeakDetect_500/xcorr_q1/Subsystem/Enabled Subsystem115 ==
  In1 : Inport
  Enable : EnablePort
  Out1 : Outport  InitialOutput=0
  wires:
  In1/1 -> Out1/1

== system PeakDetect_500/xcorr_q1/Subsystem/Enabled Subsystem116 ==
  In1 : Inport
  Enable : EnablePort
  Out1 : Outport  InitialOutput=0
  wires:
  In1/1 -> Out1/1

== system PeakDetect_500/xcorr_q1/Subsystem/Enabled Subsystem117 ==
  In1 : Inport
  Enable : EnablePort
  Out1 : Outport  InitialOutput=0
  wires:
  In1/1 -> Out1/1

== system PeakDetect_500/xcorr_q1/Subsystem/Enabled Subsystem118 ==
  In1 : Inport
  Enable : EnablePort
  Out1 : Outport  InitialOutput=0
  wires:
  In1/1 -> Out1/1

== system PeakDetect_500/xcorr_q1/Subsystem/Enabled Subsystem119 ==
  In1 : Inport
  Enable : EnablePort
  Out1 : Outport  InitialOutput=0
  wires:
  In1/1 -> Out1/1

== system PeakDetect_500/xcorr_q1/Subsystem/Enabled Subsystem120 ==
  In1 : Inport
  Enable : EnablePort
  Out1 : Outport  InitialOutput=0
  wires:
  In1/1 -> Out1/1

== system PeakDetect_500/xcorr_q1/Subsystem/Enabled Subsystem121 ==
  In1 : Inport
  Enable : EnablePort
  Out1 : Outport  InitialOutput=0
  wires:
  In1/1 -> Out1/1

== system PeakDetect_500/xcorr_q1/Subsystem/Enabled Subsystem122 ==
  In1 : Inport
  Enable : EnablePort
  Out1 : Outport  InitialOutput=0
  wires:
  In1/1 -> Out1/1

== system PeakDetect_500/xcorr_q1/Subsystem/Enabled Subsystem123 ==
  In1 : Inport
  Enable : EnablePort
  Out1 : Outport  InitialOutput=0
  wires:
  In1/1 -> Out1/1

== system PeakDetect_500/xcorr_q1/Subsystem/Enabled Subsystem124 ==
  In1 : Inport
  Enable : EnablePort
  Out1 : Outport  InitialOutput=0
  wires:
  In1/1 -> Out1/1

== system PeakDetect_500/xcorr_q1/Subsystem/Enabled Subsystem125 ==
  In1 : Inport
  Enable : EnablePort
  Out1 : Outport  InitialOutput=0
  wires:
  In1/1 -> Out1/1

== system PeakDetect_500/xcorr_q1/Subsystem/Enabled Subsystem126 ==
  In1 : Inport
  Enable : EnablePort
  Out1 : Outport  InitialOutput=0
  wires:
  In1/1 -> Out1/1

== system PeakDetect_500/xcorr_q1/Subsystem/Enabled Subsystem127 ==
  In1 : Inport
  Enable : EnablePort
  Out1 : Outport  InitialOutput=0
  wires:
  In1/1 -> Out1/1

== system PeakDetect_500/xcorr_q1/Subsystem/Enabled Subsystem128 ==
  In1 : Inport
  Enable : EnablePort
  Out1 : Outport  InitialOutput=0
  wires:
  In1/1 -> Out1/1

== system PeakDetect_500/xcorr_q1/Subsystem/Enabled Subsystem129 ==
  In1 : Inport
  Enable : EnablePort
  Out1 : Outport  InitialOutput=0
  wires:
  In1/1 -> Out1/1

== system PeakDetect_500/xcorr_q1/Subsystem/Enabled Subsystem130 ==
  In1 : Inport
  Enable : EnablePort
  Out1 : Outport  InitialOutput=0
  wires:
  In1/1 -> Out1/1

== system PeakDetect_500/xcorr_q1/Subsystem/Enabled Subsystem131 ==
  In1 : Inport
  Enable : EnablePort
  Out1 : Outport  InitialOutput=0
  wires:
  In1/1 -> Out1/1

== system PeakDetect_500/xcorr_q1/Subsystem/Enabled Subsystem132 ==
  In1 : Inport
  Enable : EnablePort
  Out1 : Outport  InitialOutput=0
  wires:
  In1/1 -> Out1/1

== system PeakDetect_500/xcorr_q1/Subsystem/Enabled Subsystem133 ==
  In1 : Inport
  Enable : EnablePort
  Out1 : Outport  InitialOutput=0
  wires:
  In1/1 -> Out1/1

== system PeakDetect_500/xcorr_q1/Subsystem/Enabled Subsystem134 ==
  In1 : Inport
  Enable : EnablePort
  Out1 : Outport  InitialOutput=0
  wires:
  In1/1 -> Out1/1

== system PeakDetect_500/xcorr_q1/Subsystem/Enabled Subsystem135 ==
  In1 : Inport
  Enable : EnablePort
  Out1 : Outport  InitialOutput=0
  wires:
  In1/1 -> Out1/1

== system PeakDetect_500/xcorr_q1/Subsystem/Enabled Subsystem136 ==
  In1 : Inport
  Enable : EnablePort
  Out1 : Outport  InitialOutput=0
  wires:
  In1/1 -> Out1/1

== system PeakDetect_500/xcorr_q1/Subsystem/Enabled Subsystem137 ==
  In1 : Inport
  Enable : EnablePort
  Out1 : Outport  InitialOutput=0
  wires:
  In1/1 -> Out1/1

== system PeakDetect_500/xcorr_q1/Subsystem/Enabled Subsystem138 ==
  In1 : Inport
  Enable : EnablePort
  Out1 : Outport  InitialOutput=0
  wires:
  In1/1 -> Out1/1

== system PeakDetect_500/xcorr_q1/Subsystem/Enabled Subsystem139 ==
  In1 : Inport
  Enable : EnablePort
  Out1 : Outport  InitialOutput=0
  wires:
  In1/1 -> Out1/1

== system PeakDetect_500/xcorr_q1/Subsystem/Enabled Subsystem140 ==
  In1 : Inport
  Enable : EnablePort
  Out1 : Outport  InitialOutput=0
  wires:
  In1/1 -> Out1/1

== system PeakDetect_500/xcorr_q1/Subsystem/Enabled Subsystem141 ==
  In1 : Inport
  Enable : EnablePort
  Out1 : Outport  InitialOutput=0
  wires:
  In1/1 -> Out1/1

== system PeakDetect_500/xcorr_q1/Subsystem/Enabled Subsystem142 ==
  In1 : Inport
  Enable : EnablePort
  Out1 : Outport  InitialOutput=0
  wires:
  In1/1 -> Out1/1

== system PeakDetect_500/xcorr_q1/Subsystem/Enabled Subsystem143 ==
  In1 : Inport
  Enable : EnablePort
  Out1 : Outport  InitialOutput=0
  wires:
  In1/1 -> Out1/1

== system PeakDetect_500/xcorr_q1/Subsystem/Enabled Subsystem144 ==
  In1 : Inport
  Enable : EnablePort
  Out1 : Outport  InitialOutput=0
  wires:
  In1/1 -> Out1/1

== system PeakDetect_500/xcorr_q1/Subsystem/Enabled Subsystem145 ==
  In1 : Inport
  Enable : EnablePort
  Out1 : Outport  InitialOutput=0
  wires:
  In1/1 -> Out1/1

== system PeakDetect_500/xcorr_q1/Subsystem/Enabled Subsystem146 ==
  In1 : Inport
  Enable : EnablePort
  Out1 : Outport  InitialOutput=0
  wires:
  In1/1 -> Out1/1

== system PeakDetect_500/xcorr_q1/Subsystem/Enabled Subsystem147 ==
  In1 : Inport
  Enable : EnablePort
  Out1 : Outport  InitialOutput=0
  wires:
  In1/1 -> Out1/1

== system PeakDetect_500/xcorr_q1/Subsystem/Enabled Subsystem148 ==
  In1 : Inport
  Enable : EnablePort
  Out1 : Outport  InitialOutput=0
  wires:
  In1/1 -> Out1/1

== system PeakDetect_500/xcorr_q1/Subsystem/Enabled Subsystem149 ==
  In1 : Inport
  Enable : EnablePort
  Out1 : Outport  InitialOutput=0
  wires:
  In1/1 -> Out1/1

== system PeakDetect_500/xcorr_q1/Subsystem/Enabled Subsystem150 ==
  In1 : Inport
  Enable : EnablePort
  Out1 : Outport  InitialOutput=0
  wires:
  In1/1 -> Out1/1

== system PeakDetect_500/xcorr_q1/Subsystem/Enabled Subsystem151 ==
  In1 : Inport
  Enable : EnablePort
  Out1 : Outport  InitialOutput=0
  wires:
  In1/1 -> Out1/1

== system PeakDetect_500/xcorr_q1/Subsystem/Enabled Subsystem152 ==
  In1 : Inport
  Enable : EnablePort
  Out1 : Outport  InitialOutput=0
  wires:
  In1/1 -> Out1/1

== system PeakDetect_500/xcorr_q1/Subsystem/Enabled Subsystem153 ==
  In1 : Inport
  Enable : EnablePort
  Out1 : Outport  InitialOutput=0
  wires:
  In1/1 -> Out1/1

== system PeakDetect_500/xcorr_q1/Subsystem/Enabled Subsystem154 ==
  In1 : Inport
  Enable : EnablePort
  Out1 : Outport  InitialOutput=0
  wires:
  In1/1 -> Out1/1

== system PeakDetect_500/xcorr_q1/Subsystem/Enabled Subsystem155 ==
  In1 : Inport
  Enable : EnablePort
  Out1 : Outport  InitialOutput=0
  wires:
  In1/1 -> Out1/1

== system PeakDetect_500/xcorr_q1/Subsystem/Enabled Subsystem156 ==
  In1 : Inport
  Enable : EnablePort
  Out1 : Outport  InitialOutput=0
  wires:
  In1/1 -> Out1/1

== system PeakDetect_500/xcorr_q1/Subsystem/Enabled Subsystem157 ==
  In1 : Inport
  Enable : EnablePort
  Out1 : Outport  InitialOutput=0
  wires:
  In1/1 -> Out1/1

== system PeakDetect_500/xcorr_q1/Subsystem/Enabled Subsystem158 ==
  In1 : Inport
  Enable : EnablePort
  Out1 : Outport  InitialOutput=0
  wires:
  In1/1 -> Out1/1

== system PeakDetect_500/xcorr_q1/Subsystem/Enabled Subsystem159 ==
  In1 : Inport
  Enable : EnablePort
  Out1 : Outport  InitialOutput=0
  wires:
  In1/1 -> Out1/1

== system PeakDetect_500/xcorr_q1/Subsystem/Enabled Subsystem160 ==
  In1 : Inport
  Enable : EnablePort
  Out1 : Outport  InitialOutput=0
  wires:
  In1/1 -> Out1/1

== system PeakDetect_500/xcorr_q1/Subsystem/Enabled Subsystem161 ==
  In1 : Inport
  Enable : EnablePort
  Out1 : Outport  InitialOutput=0
  wires:
  In1/1 -> Out1/1

== system PeakDetect_500/xcorr_q1/Subsystem/Enabled Subsystem162 ==
  In1 : Inport
  Enable : EnablePort
  Out1 : Outport  InitialOutput=0
  wires:
  In1/1 -> Out1/1

== system PeakDetect_500/xcorr_q1/Subsystem/Enabled Subsystem163 ==
  In1 : Inport
  Enable : EnablePort
  Out1 : Outport  InitialOutput=0
  wires:
  In1/1 -> Out1/1

== system PeakDetect_500/xcorr_q1/Subsystem/Enabled Subsystem164 ==
  In1 : Inport
  Enable : EnablePort
  Out1 : Outport  InitialOutput=0
  wires:
  In1/1 -> Out1/1

== system PeakDetect_500/xcorr_q1/Subsystem/Enabled Subsystem165 ==
  In1 : Inport
  Enable : EnablePort
  Out1 : Outport  InitialOutput=0
  wires:
  In1/1 -> Out1/1

== system PeakDetect_500/xcorr_q1/Subsystem/Enabled Subsystem166 ==
  In1 : Inport
  Enable : EnablePort
  Out1 : Outport  InitialOutput=0
  wires:
  In1/1 -> Out1/1

== system PeakDetect_500/xcorr_q1/Subsystem/Enabled Subsystem167 ==
  In1 : Inport
  Enable : EnablePort
  Out1 : Outport  InitialOutput=0
  wires:
  In1/1 -> Out1/1

== system PeakDetect_500/xcorr_q1/Subsystem/Enabled Subsystem168 ==
  In1 : Inport
  Enable : EnablePort
  Out1 : Outport  InitialOutput=0
  wires:
  In1/1 -> Out1/1

== system PeakDetect_500/xcorr_q1/Subsystem/Enabled Subsystem169 ==
  In1 : Inport
  Enable : EnablePort
  Out1 : Outport  InitialOutput=0
  wires:
  In1/1 -> Out1/1

== system PeakDetect_500/xcorr_q1/Subsystem/Enabled Subsystem170 ==
  In1 : Inport
  Enable : EnablePort
  Out1 : Outport  InitialOutput=0
  wires:
  In1/1 -> Out1/1

== system PeakDetect_500/xcorr_q1/Subsystem/Enabled Subsystem171 ==
  In1 : Inport
  Enable : EnablePort
  Out1 : Outport  InitialOutput=0
  wires:
  In1/1 -> Out1/1

== system PeakDetect_500/xcorr_q1/Subsystem/Enabled Subsystem172 ==
  In1 : Inport
  Enable : EnablePort
  Out1 : Outport  InitialOutput=0
  wires:
  In1/1 -> Out1/1

== system PeakDetect_500/xcorr_q1/Subsystem/Enabled Subsystem173 ==
  In1 : Inport
  Enable : EnablePort
  Out1 : Outport  InitialOutput=0
  wires:
  In1/1 -> Out1/1

== system PeakDetect_500/xcorr_q1/Subsystem/Enabled Subsystem174 ==
  In1 : Inport
  Enable : EnablePort
  Out1 : Outport  InitialOutput=0
  wires:
  In1/1 -> Out1/1

== system PeakDetect_500/xcorr_q1/Subsystem/Enabled Subsystem175 ==
  In1 : Inport
  Enable : EnablePort
  Out1 : Outport  InitialOutput=0
  wires:
  In1/1 -> Out1/1

== system PeakDetect_500/xcorr_q1/Subsystem/Enabled Subsystem176 ==
  In1 : Inport
  Enable : EnablePort
  Out1 : Outport  InitialOutput=0
  wires:
  In1/1 -> Out1/1

== system PeakDetect_500/xcorr_q1/Subsystem/Enabled Subsystem177 ==
  In1 : Inport
  Enable : EnablePort
  Out1 : Outport  InitialOutput=0
  wires:
  In1/1 -> Out1/1

== system PeakDetect_500/xcorr_q1/Subsystem/Enabled Subsystem178 ==
  In1 : Inport
  Enable : EnablePort
  Out1 : Outport  InitialOutput=0
  wires:
  In1/1 -> Out1/1

== system PeakDetect_500/xcorr_q1/Subsystem/Enabled Subsystem179 ==
  In1 : Inport
  Enable : EnablePort
  Out1 : Outport  InitialOutput=0
  wires:
  In1/1 -> Out1/1

== system PeakDetect_500/xcorr_q1/Subsystem/Enabled Subsystem180 ==
  In1 : Inport
  Enable : EnablePort
  Out1 : Outport  InitialOutput=0
  wires:
  In1/1 -> Out1/1

== system PeakDetect_500/xcorr_q1/Subsystem/Enabled Subsystem181 ==
  In1 : Inport
  Enable : EnablePort
  Out1 : Outport  InitialOutput=0
  wires:
  In1/1 -> Out1/1

== system PeakDetect_500/xcorr_q1/Subsystem/Enabled Subsystem182 ==
  In1 : Inport
  Enable : EnablePort
  Out1 : Outport  InitialOutput=0
  wires:
  In1/1 -> Out1/1

== system PeakDetect_500/xcorr_q1/Subsystem/Enabled Subsystem183 ==
  In1 : Inport
  Enable : EnablePort
  Out1 : Outport  InitialOutput=0
  wires:
  In1/1 -> Out1/1

== system PeakDetect_500/xcorr_q1/Subsystem/Enabled Subsystem184 ==
  In1 : Inport
  Enable : EnablePort
  Out1 : Outport  InitialOutput=0
  wires:
  In1/1 -> Out1/1

== system PeakDetect_500/xcorr_q1/Subsystem/Enabled Subsystem185 ==
  In1 : Inport
  Enable : EnablePort
  Out1 : Outport  InitialOutput=0
  wires:
  In1/1 -> Out1/1

== system PeakDetect_500/xcorr_q1/Subsystem/Enabled Subsystem186 ==
  In1 : Inport
  Enable : EnablePort
  Out1 : Outport  InitialOutput=0
  wires:
  In1/1 -> Out1/1

== system PeakDetect_500/xcorr_q1/Subsystem/Enabled Subsystem187 ==
  In1 : Inport
  Enable : EnablePort
  Out1 : Outport  InitialOutput=0
  wires:
  In1/1 -> Out1/1

== system PeakDetect_500/xcorr_q1/Subsystem/Enabled Subsystem188 ==
  In1 : Inport
  Enable : EnablePort
  Out1 : Outport  InitialOutput=0
  wires:
  In1/1 -> Out1/1

== system PeakDetect_500/xcorr_q1/Subsystem/Enabled Subsystem189 ==
  In1 : Inport
  Enable : EnablePort
  Out1 : Outport  InitialOutput=0
  wires:
  In1/1 -> Out1/1

== system PeakDetect_500/xcorr_q1/Subsystem/Enabled Subsystem190 ==
  In1 : Inport
  Enable : EnablePort
  Out1 : Outport  InitialOutput=0
  wires:
  In1/1 -> Out1/1

== system PeakDetect_500/xcorr_q1/Subsystem/Enabled Subsystem191 ==
  In1 : Inport
  Enable : EnablePort
  Out1 : Outport  InitialOutput=0
  wires:
  In1/1 -> Out1/1

== system PeakDetect_500/xcorr_q1/Subsystem/Enabled Subsystem192 ==
  In1 : Inport
  Enable : EnablePort
  Out1 : Outport  InitialOutput=0
  wires:
  In1/1 -> Out1/1

== system PeakDetect_500/xcorr_q1/Subsystem/Enabled Subsystem193 ==
  In1 : Inport
  Enable : EnablePort
  Out1 : Outport  InitialOutput=0
  wires:
  In1/1 -> Out1/1

== system PeakDetect_500/xcorr_q1/Subsystem/Enabled Subsystem194 ==
  In1 : Inport
  Enable : EnablePort
  Out1 : Outport  InitialOutput=0
  wires:
  In1/1 -> Out1/1

== system PeakDetect_500/xcorr_q1/Subsystem/Enabled Subsystem195 ==
  In1 : Inport
  Enable : EnablePort
  Out1 : Outport  InitialOutput=0
  wires:
  In1/1 -> Out1/1

== system PeakDetect_500/xcorr_q1/Subsystem/Enabled Subsystem196 ==
  In1 : Inport
  Enable : EnablePort
  Out1 : Outport  InitialOutput=0
  wires:
  In1/1 -> Out1/1

== system PeakDetect_500/xcorr_q1/Subsystem/Enabled Subsystem197 ==
  In1 : Inport
  Enable : EnablePort
  Out1 : Outport  InitialOutput=0
  wires:
  In1/1 -> Out1/1

== system PeakDetect_500/xcorr_q1/Subsystem/Enabled Subsystem198 ==
  In1 : Inport
  Enable : EnablePort
  Out1 : Outport  InitialOutput=0
  wires:
  In1/1 -> Out1/1

== system PeakDetect_500/xcorr_q1/Subsystem/Enabled Subsystem199 ==
  In1 : Inport
  Enable : EnablePort
  Out1 : Outport  InitialOutput=0
  wires:
  In1/1 -> Out1/1

== system PeakDetect_500/xcorr_q1/Subsystem/Enabled Subsystem200 ==
  In1 : Inport
  Enable : EnablePort
  Out1 : Outport  InitialOutput=0
  wires:
  In1/1 -> Out1/1
